simulink model "PLANTAFISICA"  (R2024a)
settings: Solver=VariableStepAuto  StartTime=0.0  StopTime=60  RelTol=1e-3
settings Model: Creator=VICTUS  LastModifiedBy=VICTUS

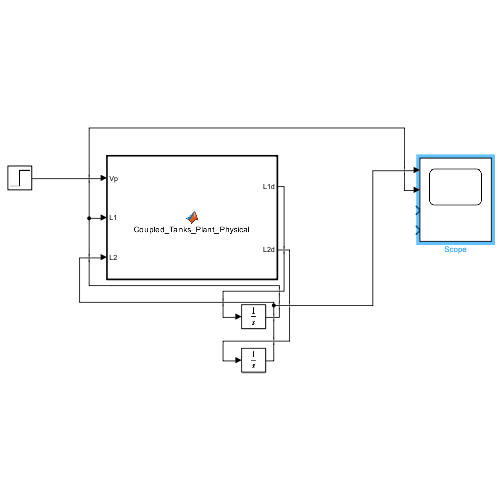
[thumbnail: Simulink's stored preview of the top-level diagram]
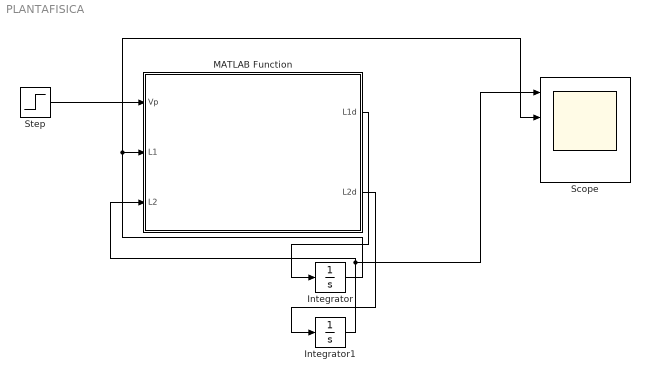
== system PLANTAFISICA ==
  Integrator : Integrator
  Integrator1 : Integrator
  MATLAB Function : MATLAB Function  TreatAsAtomicUnit=on
  Scope : Scope  NumInputPorts=4
  Step : Step  Time=0  Before=0.1  After=13.44  SampleTime=0
  wires:
  Integrator/1 -> Scope/2, MATLAB Function/2(L1)
  MATLAB Function/2(L2d) -> Integrator1/1
  MATLAB Function/1(L1d) -> Integrator/1
  Integrator1/1 -> Scope/1, MATLAB Function/3(L2)
  Step/1 -> MATLAB Function/1(Vp)

== matlab function PLANTAFISICA/MATLAB Function ==
  data: Vp input; L1d output; L2d output; L1 input; L2 input
function [L1d, L2d] = Coupled_Tanks_Plant_Physical(Vp,L1, L2)
% Modelo no lineal simplificado de tanques acoplados Quanser

dt1 = 4.445; dt2 = 4.445;
d01 = 0.635; d02 = 0.47625;
At1 = pi*(dt1^2)/4;  At2 = pi*(dt2^2)/4;
Ao1 = pi*(d01^2)/4;  Ao2 = pi*(d02^2)/4;
Kp = 3.3;  g = 981;


Fin = Kp * Vp;
Fout1 = Ao1 * sqrt(2*g*L1);
Fout2 = Ao2 * sqrt(2*g*L2);
F12 = Fout1;

L1d = (Fin - Fout1) / At1;
L2d = (F12 - Fout2) / At2;
end
